simulink model "AssemblyVero_R2019a"  (R2019a)
settings: Solver=VariableStepAuto  StartTime=0.0  StopTime=10  RelTol=1e-3
model workspace: external: MAT-File F:\College\Semester_9\GP\231123\231123\AssemblyVero_DataFile.mat (data not in the file)
undefined symbols (not defined in the file or in its folder): smiData, X, Y, Z
libraries: sm_lib x378, nesl_utility x17, simulink x4, sldrtlib x1
(part 1 of 7)
settings Model: OrderedModelArguments=off  Creator=user  LastModifiedBy=user

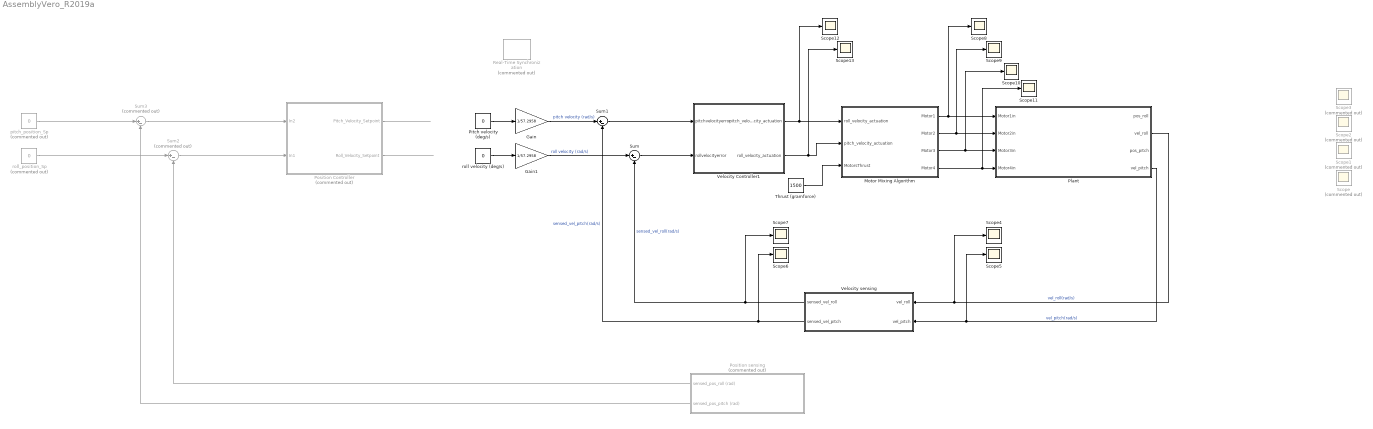
== system AssemblyVero_R2019a ==
  Gain : Gain  Gain=1/57.2958
  Gain1 : Gain  Gain=1/57.2958
  Motor Mixing Algorithm : Subsystem
  Pitch velocity (deg/s) : Constant  Value=0
  Plant : Subsystem
  Position Controller : Subsystem  Commented=on
  Position sensing : Subsystem  Commented=on
  Real-Time Synchronization : sldrtlib/Real-Time Synchronization  Commented=on  SampleTime=0.1  MaxMissedTicks=10  ShowMissedTicks=off  YieldWhenWaiting=off
  Scope{,1..3} (4 alike) : Scope  Commented=on
  Scope{4..13} (10 alike) : Scope
  Sum : Sum  Inputs=|+-
  Sum1 : Sum  Inputs=|+-
  Sum2 : Sum  Commented=on  Inputs=|+-
  Sum3 : Sum  Commented=on  Inputs=|+-
  Thrust (gramforce) : Constant  Value=1500
  Velocity Controller1 : Subsystem
  Velocity sensing : Subsystem
  pitch_position_Sp : Constant  Commented=on  Value=0
  roll velocity (deg/s) : Constant  Value=0
  roll_position_Sp : Constant  Commented=on  Value=0
  wires:
  Velocity sensing/1(sensed_vel_roll) -> Sum/2, Scope7/1  "sensed_vel_roll(rad/s)"
  Sum/1 -> Velocity Controller1/2(rollvelocityerror)
  Sum1/1 -> Velocity Controller1/1(pitchvelocityerror)
  Velocity sensing/2(sensed_vel_pitch) -> Scope6/1, Sum1/2  "sensed_vel_pitch(rad/s)"
  Position Controller/2(Roll_Velocity_Setpoint) -> ?
  Position Controller/1(Pitch_Velocity_Setpoint) -> ?
  Motor Mixing Algorithm/2(Motor2) -> Scope9/1, Plant/2(Motor2in)
  Motor Mixing Algorithm/3(Motor3) -> Scope10/1, Plant/3(Motor3in)
  Motor Mixing Algorithm/4(Motor4) -> Scope11/1, Plant/4(Motor4in)
  pitch_position_Sp/1 -> Sum3/1
  roll_position_Sp/1 -> Sum2/1
  Position sensing/2(sensed_pos_pitch (rad)) -> Sum3/2
  Sum3/1 -> Position Controller/1(In2)
  Sum2/1 -> Position Controller/2(In1)
  Position sensing/1(sensed_pos_roll (rad)) -> Sum2/2
  ? -> Scope/1  "vel_pitch"
  ? -> Scope1/1  "vel_roll"
  ? -> Scope2/1  "pos_pitch"
  ? -> Scope3/1  "pos_roll"
  Thrust (gramforce)/1 -> Motor Mixing Algorithm/3(MotorsThrust)
  roll velocity (deg/s)/1 -> Gain1/1
  Pitch velocity (deg/s)/1 -> Gain/1
  Gain/1 -> Sum1/1  "pitch velocity (rad/s)"
  Gain1/1 -> Sum/1  "roll velocity (rad/s)"
  Plant/2(vel_roll) -> Scope4/1, Velocity sensing/1(vel_roll)  "vel_roll(rad/s)"
  Plant/4(vel_pitch) -> Scope5/1, Velocity sensing/2(vel_pitch)  "vel_pitch(rad/s)"
  Motor Mixing Algorithm/1(Motor1) -> Scope8/1, Plant/1(Motor1in)
  Velocity Controller1/1(pitch_velocity_actuation) -> Scope12/1, Motor Mixing Algorithm/1(roll_velocity_actuation)
  Velocity Controller1/2(roll_velocity_actuation) -> Scope13/1, Motor Mixing Algorithm/2(pitch_velocity_actuation)

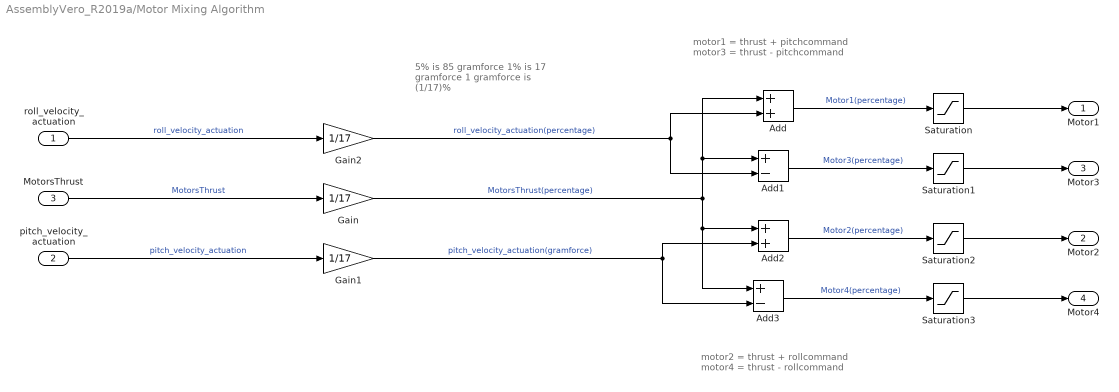
== system AssemblyVero_R2019a/Motor Mixing Algorithm ==
  note: 5% is 85 gramforce
      | 1% is 17 gramforce
      | 1 gramforce is (1/17)%
  note: motor1 = thrust + pitchcommand
      | motor3 = thrust - pitchcommand
  note: motor2 = thrust + rollcommand
      | motor4 = thrust - rollcommand
  roll_velocity_actuation : Inport
  pitch_velocity_actuation : Inport  Port=2
  MotorsThrust : Inport  Port=3
  Add : Sum
  Add1 : Sum  Inputs=+-
  Add2 : Sum
  Add3 : Sum  Inputs=+-
  Gain : Gain  Gain=1/17
  Gain1 : Gain  Gain=1/17
  Gain2 : Gain  Gain=1/17
  Saturation{,1..3} (4 alike) : Saturate  UpperLimit=100  LowerLimit=0
  Motor1 : Outport
  Motor2 : Outport  Port=2
  Motor3 : Outport  Port=3
  Motor4 : Outport  Port=4
  wires:
  Gain2/1 -> Add1/2, Add/2  "roll_velocity_actuation(percentage)"
  Add/1 -> Saturation/1  "Motor1(percentage)"
  Add1/1 -> Saturation1/1  "Motor3(percentage)"
  Add3/1 -> Saturation3/1  "Motor4(percentage)"
  Add2/1 -> Saturation2/1  "Motor2(percentage)"
  Gain1/1 -> Add3/2, Add2/2  "pitch_velocity_actuation(gramforce)"
  MotorsThrust/1 -> Gain/1  "MotorsThrust"
  Gain/1 -> Add3/1, Add2/1, Add1/1, Add/1  "MotorsThrust(percentage)"
  roll_velocity_actuation/1 -> Gain2/1  "roll_velocity_actuation"
  pitch_velocity_actuation/1 -> Gain1/1  "pitch_velocity_actuation"
  Saturation/1 -> Motor1/1
  Saturation1/1 -> Motor3/1
  Saturation2/1 -> Motor2/1
  Saturation3/1 -> Motor4/1

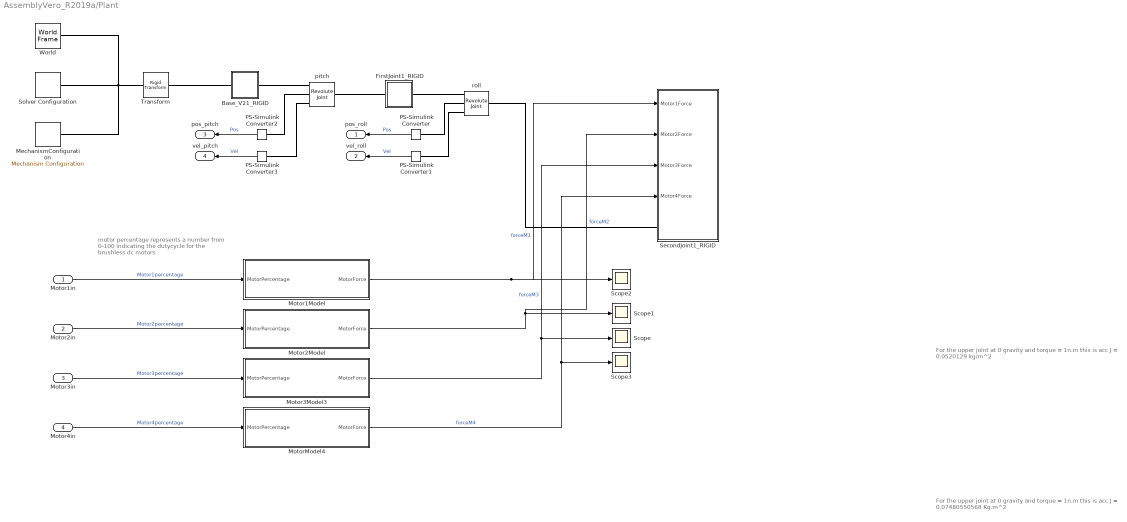
== system AssemblyVero_R2019a/Plant ==
  note: motor percentage represents a number from 0-100 indicating the dutycycle for the brushless dc motors
  note: For the upper joint at 0 gravity and torque = 1n.m this is acc
      | J = 0.07480550568 Kg.m^2
  note: For the upper joint at 0 gravity and torque = 1n.m this is acc
      | J = 0.0520129 kg/m^2
  Motor1in : Inport
  Motor2in : Inport  Port=2
  Motor3in : Inport  Port=3
  Motor4in : Inport  Port=4
  Base_V21_RIGID : Subsystem
  FirstJoint1_RIGID : Subsystem
  MechanismConfiguration : sm_lib/Utilities/Mechanism Configuration  UniformGravity=Constant  GravityVector=[0 0 -9.80665]  GravityVectorUnits=m/s^2  GravityUnits=m/s^2  LinearizationDelta=0.001  JointModeTransitionNonlinearIterations=2
  Motor1Model : Subsystem
  Motor2Model : Subsystem
  Motor3Model3 : Subsystem
  MotorModel4 : Subsystem
  PS-Simulink Converter{,1..3} (4 alike) : nesl_utility/PS-Simulink Converter  PhysicalDomain=network_engine_domain  SubClassName=ps_output  LeftPortType=input  RightPortType=output  PseudoPeriodic=off  Frequencies=[]  Unit=inherit  AffineConversion=off
  Scope{,1..3} (4 alike) : Scope
  SecondJoint1_RIGID : Subsystem
  Solver Configuration : nesl_utility/Solver Configuration  PhysicalDomain=network_engine_domain  SubClassName=solver  LeftPortType=input  RightPortType=generic  Tones=[]  Harmonics=[]  SimulateNoise=off  Profile=off  UseLocalSampling=off  EnableSwitchedLinearOptims=on  FrequencyDomain=off  UseCCode=off  RelTol=0.001  AbsTol=1e-06  MinStep=1e-09  ToWorkspace=off  RevertToSquareIcSolve=off  NumHomotopyIterations=100  PhasorMode=off  PhasorModeNumHarmonics=1  DoDC=off  ResidualTolerance=1e-09  UseLocalSolver=off  LocalSolverChoice=NE_BACKWARD_EULER_ADVANCER  LocalSolverSampleTime=0.001  DoFixedCost=off  MaxNonlinIter=3  MaxModeIter=2  ComputeImpulses=off  ImpulseIterations=2  LinearAlgebra=auto  EquationFormulation=NE_TIME_EF  DelaysMemoryBudget=1024  AutomaticFiltering=on  FilteringTimeConstant=0.001  PartitionStorageMethod=AS_NEEDED  PartitionMemoryBudget=1024  PartitionMethod=ROBUST
  Transform : sm_lib/Frames and Transforms/Rigid Transform  TranslationMethod=Cartesian  TranslationStandardOffset=0  TranslationLengthUnit=mm  TranslationStandardAxis=+Z  TranslationCartesianOffset=smiData.RigidTransform(123).translation  TranslationROffset=0  TranslationROffsetUnits=m  TranslationZOffset=0  TranslationZOffsetUnits=m  TranslationThetaOffset=0  TranslationThetaOffsetUnits=deg  RotationMethod=ArbitraryAxis  RotationAngleUnits=rad  RotationStandardAxis=+Z  RotationAngle=smiData.RigidTransform(123).angle  RotationArbitraryAxis=smiData.RigidTransform(123).axis  FollAlignAxisA=+X  BaseAlignAxisA=+Y  FollAlignAxisB=+Y  BaseAlignAxisB=+Z  RotationSequenceAxes=FollowerAxes  RotationSequence=XYX  RotationSequenceAngles=[0 0 0]  RotationSequenceAnglesUnits=deg  RotationMatrix=[1 0 0; 0 1 0; 0 0 1]
  World : sm_lib/Frames and Transforms/World Frame
  pitch : sm_lib/Joints/Revolute Joint  JointMode=Normal  SenseConstraintForce=off  SenseConstraintForceX=off  SenseConstraintForceY=off  SenseConstraintForceZ=off  SenseConstraintTorque=off  SenseConstraintTorqueX=off  SenseConstraintTorqueY=off  SenseConstraintTorqueZ=off  SenseTotalForce=off  SenseTotalForceX=off  SenseTotalForceY=off  SenseTotalForceZ=off  SenseTotalTorque=off  SenseTotalTorqueX=off  SenseTotalTorqueY=off  SenseTotalTorqueZ=off  CompositeWrenchDir=FollowerOnBase  CompositeWrenchFrame=BaseFrame  EquilibriumPosition=0  EquilibriumPositionUnits=deg  SpringStiffness=0  SpringStiffnessUnits=N*m/deg  DampingCoefficient=0  DampingCoefficientUnits=N*m/(deg/s)  TorqueActuationMode=NoTorque  MotionActuationMode=ComputedMotion  SensePosition=on  SenseVelocity=on  SenseAcceleration=off  SenseTorqueForce=off  SenseLowerLimitTorqueForce=off  SenseUpperLimitTorqueForce=off  LowerLimitSpecify=on  LowerLimitBound=smiData.RevoluteJoint(1).Rz.Pos -35  LowerLimitBoundUnits=deg  LowerLimitStiffness=1e4  LowerLimitStiffnessUnits=N*m/deg  LowerLimitDamping=10  LowerLimitDampingUnits=N*m/(deg/s)  LowerLimitTransitionRegionWidth=0.1  LowerLimitTransitionRegionWidthUnits=deg  UpperLimitSpecify=on  UpperLimitBound=smiData.RevoluteJoint(1).Rz.Pos+35  UpperLimitBoundUnits=deg  UpperLimitStiffness=1e4  UpperLimitStiffnessUnits=N*m/deg  UpperLimitDamping=10  UpperLimitDampingUnits=N*m/(deg/s)  UpperLimitTransitionRegionWidth=0.1  UpperLimitTransitionRegionWidthUnits=deg  PositionTargetSpecify=on  PositionTargetPriority=Low  PositionTargetValue=smiData.RevoluteJoint(1).Rz.Pos  PositionTargetValueUnits=deg  VelocityTargetSpecify=off  VelocityTargetPriority=High  VelocityTargetValue=0  VelocityTargetValueUnits=deg/s
  roll : sm_lib/Joints/Revolute Joint  JointMode=Normal  SenseConstraintForce=off  SenseConstraintForceX=off  SenseConstraintForceY=off  SenseConstraintForceZ=off  SenseConstraintTorque=off  SenseConstraintTorqueX=off  SenseConstraintTorqueY=off  SenseConstraintTorqueZ=off  SenseTotalForce=off  SenseTotalForceX=off  SenseTotalForceY=off  SenseTotalForceZ=off  SenseTotalTorque=off  SenseTotalTorqueX=off  SenseTotalTorqueY=off  SenseTotalTorqueZ=off  CompositeWrenchDir=FollowerOnBase  CompositeWrenchFrame=BaseFrame  EquilibriumPosition=0  EquilibriumPositionUnits=deg  SpringStiffness=0  SpringStiffnessUnits=N*m/deg  DampingCoefficient=0  DampingCoefficientUnits=N*m/(deg/s)  TorqueActuationMode=NoTorque  MotionActuationMode=ComputedMotion  SensePosition=on  SenseVelocity=on  SenseAcceleration=off  SenseTorqueForce=off  SenseLowerLimitTorqueForce=off  SenseUpperLimitTorqueForce=off  LowerLimitSpecify=on  LowerLimitBound=smiData.RevoluteJoint(2).Rz.Pos-35  LowerLimitBoundUnits=deg  LowerLimitStiffness=1e4  LowerLimitStiffnessUnits=N*m/deg  LowerLimitDamping=10  LowerLimitDampingUnits=N*m/(deg/s)  LowerLimitTransitionRegionWidth=0.1  LowerLimitTransitionRegionWidthUnits=deg  UpperLimitSpecify=on  UpperLimitBound=smiData.RevoluteJoint(2).Rz.Pos+35  UpperLimitBoundUnits=deg  UpperLimitStiffness=1e4  UpperLimitStiffnessUnits=N*m/deg  UpperLimitDamping=10  UpperLimitDampingUnits=N*m/(deg/s)  UpperLimitTransitionRegionWidth=0.1  UpperLimitTransitionRegionWidthUnits=deg  PositionTargetSpecify=on  PositionTargetPriority=Low  PositionTargetValue=smiData.RevoluteJoint(2).Rz.Pos  PositionTargetValueUnits=deg  VelocityTargetSpecify=on  VelocityTargetPriority=High  VelocityTargetValue=0  VelocityTargetValueUnits=deg/s
  pos_roll : Outport
  vel_roll : Outport  Port=2
  pos_pitch : Outport  Port=3
  vel_pitch : Outport  Port=4
  wires:
  Motor2Model/1(MotorForce) -> SecondJoint1_RIGID/2(Motor2Force), Scope1/1  "forceM2"
  MotorModel4/1(MotorForce) -> Scope3/1, SecondJoint1_RIGID/4(Motor4Force)  "forceM4"
  Motor3Model3/1(MotorForce) -> Scope/1, SecondJoint1_RIGID/3(Motor3Force)  "forceM3"
  Motor2in/1 -> Motor2Model/1(MotorPercentage)  "Motor2percentage"
  Motor3in/1 -> Motor3Model3/1(MotorPercentage)  "Motor3percentage"
  Motor4in/1 -> MotorModel4/1(MotorPercentage)  "Motor4percentage"
  Motor1in/1 -> Motor1Model/1(MotorPercentage)  "Motor1percentage"
  Motor1Model/1(MotorForce) -> SecondJoint1_RIGID/1(Motor1Force), Scope2/1  "forceM1"
  PS-Simulink Converter/1 -> pos_roll/1  "Pos"
  PS-Simulink Converter1/1 -> vel_roll/1  "Vel"
  PS-Simulink Converter3/1 -> vel_pitch/1  "Vel"
  PS-Simulink Converter2/1 -> pos_pitch/1  "Pos"
  connections:
  Transform/LConn1 -- World/RConn1 -- Solver Configuration/RConn1 -- MechanismConfiguration/RConn1
  Base_V21_RIGID/RConn1 -- pitch/RConn1
  roll/LConn1 -- SecondJoint1_RIGID/LConn1
  FirstJoint1_RIGID/RConn1 -- pitch/LConn1
  FirstJoint1_RIGID/LConn1 -- roll/RConn1
  Base_V21_RIGID/LConn1 -- Transform/RConn1
  roll/RConn3 -- PS-Simulink Converter1/LConn1
  roll/RConn2 -- PS-Simulink Converter/LConn1
  PS-Simulink Converter2/LConn1 -- pitch/RConn2
  pitch/RConn3 -- PS-Simulink Converter3/LConn1

== system AssemblyVero_R2019a/Position Controller ==
  In2 : Inport
  In1 : Inport  Port=2
  PID Controller : simulink/Continuous/PID Controller  Controller=PID  Form=Parallel  TimeDomain=Continuous-time  SampleTime=-1  IntegratorMethod=Forward Euler  FilterMethod=Forward Euler  ControllerParametersSource=internal  P=1  I=1  D=0  UseFilter=on  N=100  TunerSelectOption=Transfer Function Based (PID Tuner App)  InitialConditionSource=internal  InitialConditionForIntegrator=0  InitialConditionForFilter=0  DifferentiatorICPrevScaledInput=0  ExternalReset=none  TrackingMode=off  Kt=1  LimitOutput=off  UpperSaturationLimit=inf  LowerSaturationLimit=-inf  LinearizeAsGain=on  AntiWindupMode=none  Kb=1  POutMin=[]  POutMax=[]  IOutMin=[]  IOutMax=[]  DOutMin=[]  DOutMax=[]  NOutMin=[]  NOutMax=[]  SumOutMin=[]  SumOutMax=[]  SaturationOutMin=[]  SaturationOutMax=[]  PParamMin=[]  PParamMax=[]  IParamMin=[]  IParamMax=[]  DParamMin=[]  DParamMax=[]  NParamMin=[]  NParamMax=[]  KbParamMin=[]  KbParamMax=[]  KtParamMin=[]  KtParamMax=[]  KbOutMin=[]  KbOutMax=[]  KtOutMin=[]  KtOutMax=[]  IntegratorOutMin=[]  IntegratorOutMax=[]  FilterOutMin=[]  FilterOutMax=[]  SumI1OutMin=[]  SumI1OutMax=[]  SumI2OutMin=[]  SumI2OutMax=[]  SumI3OutMin=[]  SumI3OutMax=[]  SumI4OutMin=[]  SumI4OutMax=[]  SumDOutMin=[]  SumDOutMax=[]  DifferentiatorOutMin=[]  DifferentiatorOutMax=[]  FilterDiffOutCoefMin=[]  FilterDiffOutCoefMax=[]  ReciprocalOutMin=[]  ReciprocalOutMax=[]  SumDenOutMin=[]  SumDenOutMax=[]  SumNumOutMin=[]  SumNumOutMax=[]  DivideOutMin=[]  DivideOutMax=[]  IntegratorContinuousStateAttributes=''  IntegratorStateMustResolveToSignalObject=off  IntegratorRTWStateStorageClass=Auto  FilterContinuousStateAttributes=''  FilterStateMustResolveToSignalObject=off  FilterRTWStateStorageClass=Auto  ParallelPVariant=InternalParameters  IdealPVariant=Disabled  IVariant=InternalParameters  DVariant=InternalParameters  IntegratorVariant=Continuous  SatVariant=Disabled  AWVariant=Passthrough  PCopyVariant=Disabled  TRVariant=Disabled  FdbkBlocksVariant=Forward  IdealPFdbkVariant=Disabled  SatFdbkVariant=Disabled  DerivativeFilterVariant=ContFilter  NVariant=InternalParameters  NCopyVariant=Disabled  FilterICVariant=InternalICsFilter  IntegratorICVariant=InternalICs  ExternalResetVariant=Disabled  TRSumVariant=Passthrough  SumFdbkVariant=Disabled  SumVariant=Sum_PID
  PID Controller1 : simulink/Continuous/PID Controller  Controller=PID  Form=Parallel  TimeDomain=Continuous-time  SampleTime=-1  IntegratorMethod=Forward Euler  FilterMethod=Forward Euler  ControllerParametersSource=internal  P=1  I=1  D=0  UseFilter=on  N=100  TunerSelectOption=Transfer Function Based (PID Tuner App)  InitialConditionSource=internal  InitialConditionForIntegrator=0  InitialConditionForFilter=0  DifferentiatorICPrevScaledInput=0  ExternalReset=none  TrackingMode=off  Kt=1  LimitOutput=off  UpperSaturationLimit=inf  LowerSaturationLimit=-inf  LinearizeAsGain=on  AntiWindupMode=none  Kb=1  POutMin=[]  POutMax=[]  IOutMin=[]  IOutMax=[]  DOutMin=[]  DOutMax=[]  NOutMin=[]  NOutMax=[]  SumOutMin=[]  SumOutMax=[]  SaturationOutMin=[]  SaturationOutMax=[]  PParamMin=[]  PParamMax=[]  IParamMin=[]  IParamMax=[]  DParamMin=[]  DParamMax=[]  NParamMin=[]  NParamMax=[]  KbParamMin=[]  KbParamMax=[]  KtParamMin=[]  KtParamMax=[]  KbOutMin=[]  KbOutMax=[]  KtOutMin=[]  KtOutMax=[]  IntegratorOutMin=[]  IntegratorOutMax=[]  FilterOutMin=[]  FilterOutMax=[]  SumI1OutMin=[]  SumI1OutMax=[]  SumI2OutMin=[]  SumI2OutMax=[]  SumI3OutMin=[]  SumI3OutMax=[]  SumI4OutMin=[]  SumI4OutMax=[]  SumDOutMin=[]  SumDOutMax=[]  DifferentiatorOutMin=[]  DifferentiatorOutMax=[]  FilterDiffOutCoefMin=[]  FilterDiffOutCoefMax=[]  ReciprocalOutMin=[]  ReciprocalOutMax=[]  SumDenOutMin=[]  SumDenOutMax=[]  SumNumOutMin=[]  SumNumOutMax=[]  DivideOutMin=[]  DivideOutMax=[]  IntegratorContinuousStateAttributes=''  IntegratorStateMustResolveToSignalObject=off  IntegratorRTWStateStorageClass=Auto  FilterContinuousStateAttributes=''  FilterStateMustResolveToSignalObject=off  FilterRTWStateStorageClass=Auto  ParallelPVariant=InternalParameters  IdealPVariant=Disabled  IVariant=InternalParameters  DVariant=InternalParameters  IntegratorVariant=Continuous  SatVariant=Disabled  AWVariant=Passthrough  PCopyVariant=Disabled  TRVariant=Disabled  FdbkBlocksVariant=Forward  IdealPFdbkVariant=Disabled  SatFdbkVariant=Disabled  DerivativeFilterVariant=ContFilter  NVariant=InternalParameters  NCopyVariant=Disabled  FilterICVariant=InternalICsFilter  IntegratorICVariant=InternalICs  ExternalResetVariant=Disabled  TRSumVariant=Passthrough  SumFdbkVariant=Disabled  SumVariant=Sum_PID
  Transport Delay : TransportDelay  DelayTime=0.05
  Transport Delay1 : TransportDelay  DelayTime=0.05
  Pitch_Velocity_Setpoint : Outport
  Roll_Velocity_Setpoint : Outport  Port=2
  wires:
  PID Controller/1 -> Transport Delay1/1
  In2/1 -> PID Controller/1
  In1/1 -> PID Controller1/1
  PID Controller1/1 -> Transport Delay/1
  Transport Delay/1 -> Roll_Velocity_Setpoint/1
  Transport Delay1/1 -> Pitch_Velocity_Setpoint/1

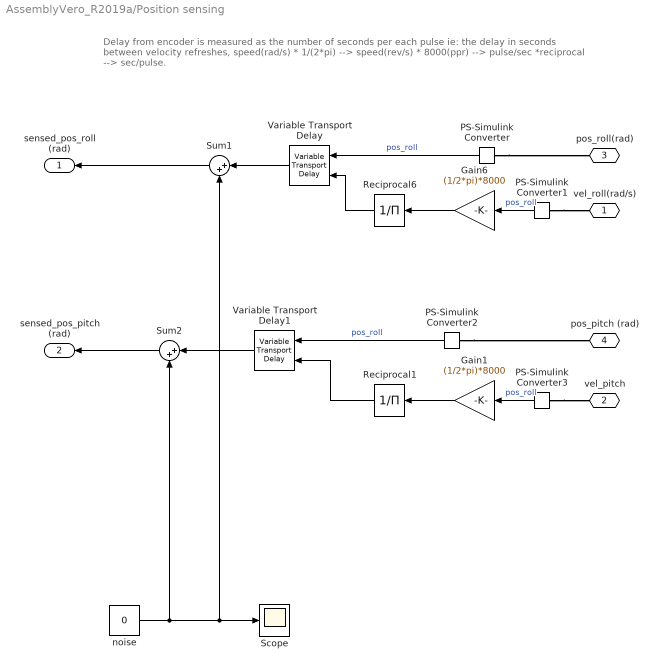
== system AssemblyVero_R2019a/Position sensing ==
  note: Delay from encoder is measured as the number of seconds per each pulse ie: the delay in seconds between velocity refreshes, speed(rad/s) * 1/(2*pi) --> speed(rev/s) * 8000(ppr) --> pulse/sec *reciprocal --> sec/pulse.
  Gain1 : Gain  Gain=(1/2*pi)*8000
  Gain6 : Gain  Gain=(1/2*pi)*8000
  PS-Simulink Converter{,1..3} (4 alike) : nesl_utility/PS-Simulink Converter  PhysicalDomain=network_engine_domain  SubClassName=ps_output  LeftPortType=input  RightPortType=output  PseudoPeriodic=off  Frequencies=[]  Unit=inherit  AffineConversion=off
  Reciprocal1 : Product  Inputs=/
  Reciprocal6 : Product  Inputs=/
  Scope : Scope
  Sum1 : Sum  Inputs=|++
  Sum2 : Sum  Inputs=|++
  Variable Transport Delay : VariableTransportDelay  VariableDelayType=Variable transport delay  MaximumDelay=0.2
  Variable Transport Delay1 : VariableTransportDelay  VariableDelayType=Variable transport delay  MaximumDelay=0.2
  noise : Constant  Value=0
  vel_roll(rad/s) : PMIOPort  Side=Left
  vel_pitch : PMIOPort  Port=2  Side=Left
  pos_roll(rad) : PMIOPort  Port=3  Side=Left
  pos_pitch (rad) : PMIOPort  Port=4  Side=Left
  sensed_pos_roll (rad) : Outport
  sensed_pos_pitch (rad) : Outport  Port=2
  wires:
  Sum1/1 -> sensed_pos_roll (rad)/1
  Reciprocal6/1 -> Variable Transport Delay/2
  Variable Transport Delay/1 -> Sum1/1
  PS-Simulink Converter/1 -> Variable Transport Delay/1  "pos_roll"
  Gain6/1 -> Reciprocal6/1
  noise/1 -> Sum2/2, Sum1/2, Scope/1
  PS-Simulink Converter1/1 -> Gain6/1  "pos_roll"
  PS-Simulink Converter3/1 -> Gain1/1  "pos_roll"
  Gain1/1 -> Reciprocal1/1
  PS-Simulink Converter2/1 -> Variable Transport Delay1/1  "pos_roll"
  Variable Transport Delay1/1 -> Sum2/1
  Reciprocal1/1 -> Variable Transport Delay1/2
  Sum2/1 -> sensed_pos_pitch (rad)/1
  connections:
  PS-Simulink Converter2/LConn1 -- pos_pitch (rad)/RConn1
  PS-Simulink Converter/LConn1 -- pos_roll(rad)/RConn1
  PS-Simulink Converter1/LConn1 -- vel_roll(rad/s)/RConn1
  PS-Simulink Converter3/LConn1 -- vel_pitch/RConn1

== system AssemblyVero_R2019a/Velocity Controller1 ==
  pitchvelocityerror : Inport
  rollvelocityerror : Inport  Port=2
  PID Controller : simulink/Continuous/PID Controller  Controller=PID  Form=Parallel  TimeDomain=Discrete-time  SampleTime=-1  IntegratorMethod=Forward Euler  FilterMethod=Forward Euler  ControllerParametersSource=internal  P=100  I=0  D=0  UseFilter=on  N=100  TunerSelectOption=Transfer Function Based (PID Tuner App)  InitialConditionSource=internal  InitialConditionForIntegrator=0  InitialConditionForFilter=0  DifferentiatorICPrevScaledInput=0  ExternalReset=none  TrackingMode=off  Kt=1  LimitOutput=off  UpperSaturationLimit=inf  LowerSaturationLimit=-inf  LinearizeAsGain=on  AntiWindupMode=none  Kb=1  POutMin=[]  POutMax=[]  IOutMin=[]  IOutMax=[]  DOutMin=[]  DOutMax=[]  NOutMin=[]  NOutMax=[]  SumOutMin=[]  SumOutMax=[]  SaturationOutMin=[]  SaturationOutMax=[]  PParamMin=[]  PParamMax=[]  IParamMin=[]  IParamMax=[]  DParamMin=[]  DParamMax=[]  NParamMin=[]  NParamMax=[]  KbParamMin=[]  KbParamMax=[]  KtParamMin=[]  KtParamMax=[]  KbOutMin=[]  KbOutMax=[]  KtOutMin=[]  KtOutMax=[]  IntegratorOutMin=[]  IntegratorOutMax=[]  FilterOutMin=[]  FilterOutMax=[]  SumI1OutMin=[]  SumI1OutMax=[]  SumI2OutMin=[]  SumI2OutMax=[]  SumI3OutMin=[]  SumI3OutMax=[]  SumI4OutMin=[]  SumI4OutMax=[]  SumDOutMin=[]  SumDOutMax=[]  DifferentiatorOutMin=[]  DifferentiatorOutMax=[]  FilterDiffOutCoefMin=[]  FilterDiffOutCoefMax=[]  ReciprocalOutMin=[]  ReciprocalOutMax=[]  SumDenOutMin=[]  SumDenOutMax=[]  SumNumOutMin=[]  SumNumOutMax=[]  DivideOutMin=[]  DivideOutMax=[]  IntegratorContinuousStateAttributes=''  IntegratorStateMustResolveToSignalObject=off  IntegratorRTWStateStorageClass=Auto  FilterContinuousStateAttributes=''  FilterStateMustResolveToSignalObject=off  FilterRTWStateStorageClass=Auto  ParallelPVariant=InternalParameters  IdealPVariant=Disabled  IVariant=InternalParameters  DVariant=InternalParameters  IntegratorVariant=Discrete  SatVariant=Disabled  AWVariant=Passthrough  PCopyVariant=Disabled  TRVariant=Disabled  FdbkBlocksVariant=Forward  IdealPFdbkVariant=Disabled  SatFdbkVariant=Disabled  DerivativeFilterVariant=ForwardEulerFilter  NVariant=InternalParameters  NCopyVariant=Disabled  FilterICVariant=InternalICsFilter  IntegratorICVariant=InternalICs  ExternalResetVariant=Disabled  TRSumVariant=Passthrough  SumFdbkVariant=Disabled  SumVariant=Sum_PID
  PID Controller1 : simulink/Continuous/PID Controller  Controller=PID  Form=Parallel  TimeDomain=Discrete-time  SampleTime=-1  IntegratorMethod=Forward Euler  FilterMethod=Forward Euler  ControllerParametersSource=internal  P=100  I=0  D=0  UseFilter=on  N=100  TunerSelectOption=Transfer Function Based (PID Tuner App)  InitialConditionSource=internal  InitialConditionForIntegrator=0  InitialConditionForFilter=0  DifferentiatorICPrevScaledInput=0  ExternalReset=none  TrackingMode=off  Kt=1  LimitOutput=off  UpperSaturationLimit=inf  LowerSaturationLimit=-inf  LinearizeAsGain=on  AntiWindupMode=none  Kb=1  POutMin=[]  POutMax=[]  IOutMin=[]  IOutMax=[]  DOutMin=[]  DOutMax=[]  NOutMin=[]  NOutMax=[]  SumOutMin=[]  SumOutMax=[]  SaturationOutMin=[]  SaturationOutMax=[]  PParamMin=[]  PParamMax=[]  IParamMin=[]  IParamMax=[]  DParamMin=[]  DParamMax=[]  NParamMin=[]  NParamMax=[]  KbParamMin=[]  KbParamMax=[]  KtParamMin=[]  KtParamMax=[]  KbOutMin=[]  KbOutMax=[]  KtOutMin=[]  KtOutMax=[]  IntegratorOutMin=[]  IntegratorOutMax=[]  FilterOutMin=[]  FilterOutMax=[]  SumI1OutMin=[]  SumI1OutMax=[]  SumI2OutMin=[]  SumI2OutMax=[]  SumI3OutMin=[]  SumI3OutMax=[]  SumI4OutMin=[]  SumI4OutMax=[]  SumDOutMin=[]  SumDOutMax=[]  DifferentiatorOutMin=[]  DifferentiatorOutMax=[]  FilterDiffOutCoefMin=[]  FilterDiffOutCoefMax=[]  ReciprocalOutMin=[]  ReciprocalOutMax=[]  SumDenOutMin=[]  SumDenOutMax=[]  SumNumOutMin=[]  SumNumOutMax=[]  DivideOutMin=[]  DivideOutMax=[]  IntegratorContinuousStateAttributes=''  IntegratorStateMustResolveToSignalObject=off  IntegratorRTWStateStorageClass=Auto  FilterContinuousStateAttributes=''  FilterStateMustResolveToSignalObject=off  FilterRTWStateStorageClass=Auto  ParallelPVariant=InternalParameters  IdealPVariant=Disabled  IVariant=InternalParameters  DVariant=InternalParameters  IntegratorVariant=Discrete  SatVariant=Disabled  AWVariant=Passthrough  PCopyVariant=Disabled  TRVariant=Disabled  FdbkBlocksVariant=Forward  IdealPFdbkVariant=Disabled  SatFdbkVariant=Disabled  DerivativeFilterVariant=ForwardEulerFilter  NVariant=InternalParameters  NCopyVariant=Disabled  FilterICVariant=InternalICsFilter  IntegratorICVariant=InternalICs  ExternalResetVariant=Disabled  TRSumVariant=Passthrough  SumFdbkVariant=Disabled  SumVariant=Sum_PID
  Transport Delay : TransportDelay  DelayTime=0.05
  Transport Delay1 : TransportDelay  DelayTime=0.05
  pitch_velocity_actuation : Outport
  roll_velocity_actuation : Outport  Port=2
  wires:
  PID Controller/1 -> Transport Delay/1  "pitch_velocity_actuation"
  pitchvelocityerror/1 -> PID Controller/1  "pitch_error(rad/s)"
  rollvelocityerror/1 -> PID Controller1/1  "roll_error(rad/s)"
  PID Controller1/1 -> Transport Delay1/1  "pitch_velocity_actuation"
  Transport Delay/1 -> pitch_velocity_actuation/1
  Transport Delay1/1 -> roll_velocity_actuation/1

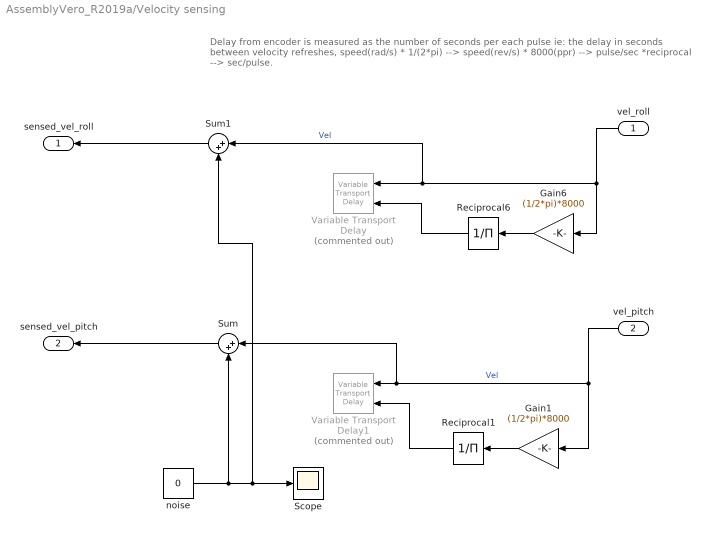
== system AssemblyVero_R2019a/Velocity sensing ==
  note: Delay from encoder is measured as the number of seconds per each pulse ie: the delay in seconds between velocity refreshes, speed(rad/s) * 1/(2*pi) --> speed(rev/s) * 8000(ppr) --> pulse/sec *reciprocal --> sec/pulse.
  vel_roll : Inport
  vel_pitch : Inport  Port=2
  Gain1 : Gain  Gain=(1/2*pi)*8000
  Gain6 : Gain  Gain=(1/2*pi)*8000
  Reciprocal1 : Product  Inputs=/
  Reciprocal6 : Product  Inputs=/
  Scope : Scope
  Sum : Sum  Inputs=|++
  Sum1 : Sum  Inputs=|++
  Variable Transport Delay : VariableTransportDelay  Commented=on  VariableDelayType=Variable transport delay  MaximumDelay=0.2
  Variable Transport Delay1 : VariableTransportDelay  Commented=on  VariableDelayType=Variable transport delay  MaximumDelay=0.2
  noise : Constant  Value=0
  sensed_vel_roll : Outport
  sensed_vel_pitch : Outport  Port=2
  wires:
  vel_roll/1 -> Gain6/1, Sum1/1, Variable Transport Delay/1  "Vel"
  Gain6/1 -> Reciprocal6/1
  Reciprocal6/1 -> Variable Transport Delay/2
  Reciprocal1/1 -> Variable Transport Delay1/2
  Gain1/1 -> Reciprocal1/1
  vel_pitch/1 -> Sum/1, Variable Transport Delay1/1, Gain1/1  "Vel"
  noise/1 -> Scope/1, Sum1/2, Sum/2
  Sum/1 -> sensed_vel_pitch/1
  Sum1/1 -> sensed_vel_roll/1
